simulink subsystem "ParachuteSpatial3DOF"  (R2023b)
settings: Solver=VariableStepAuto  StartTime=0.0  StopTime=10.0  RelTol=1e-3
undefined symbols (not defined in the file): alt
libraries: aerolibatmos2 x1, matrix_library x1, vrlib x1
settings Model: Creator=thatf  LastModifiedBy=thatf

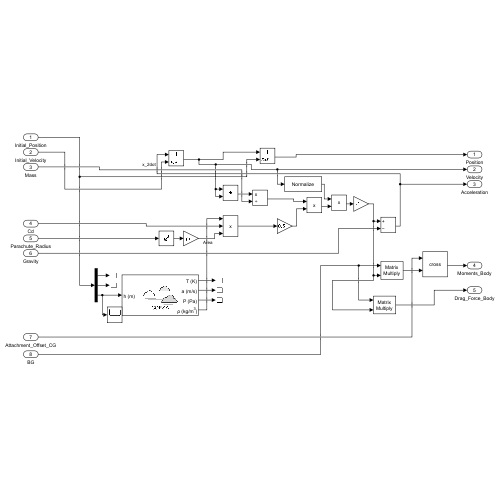
[thumbnail: Simulink's stored preview of the top-level diagram]
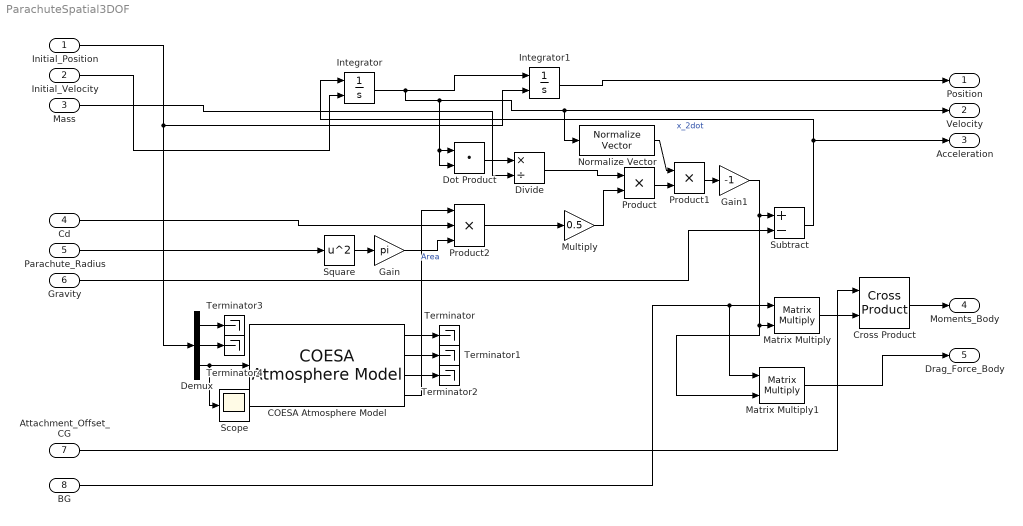
== system ParachuteSpatial3DOF ==
  Initial_Position : Inport
  Initial_Velocity : Inport  Port=2
  Mass : Inport  Port=3
  Cd : Inport  Port=4
  Parachute_Radius : Inport  Port=5
  Gravity : Inport  Port=6
  Attachment_Offset_CG : Inport  Port=7
  BG : Inport  Port=8
  COESA Atmosphere Model : aerolibatmos2/COESA Atmosphere Model  units=Metric (MKS)  spec=1976 COESA-extended U.S. Standard Atmosphere  model=Profile  profile_var=High temperature  profile_percent=1%  profile_alt=5 km (16404 ft)  envelope_var=High temperature  envelope_percent=1%  action=Warning
  Cross Product : matrix_library/Cross Product
  Demux : Demux  Outputs=3
  Divide : Product  Inputs=*/
  Dot Product : DotProduct  OutDataTypeStr=Inherit: Inherit via internal rule
  Gain : Gain  Gain=pi
  Gain1 : Gain  Gain=-1
  Integrator : Integrator  InitialConditionSource=external
  Integrator1 : Integrator  InitialConditionSource=external  InitialCondition=alt
  Matrix Multiply : Product  Multiplication=Matrix(*)
  Matrix Multiply1 : Product  Multiplication=Matrix(*)
  Multiply : Gain  Gain=0.5
  Normalize Vector : vrlib/Utilities/Normalize Vector  maxzero=0
  Product : Product
  Product1 : Product
  Product2 : Product  Inputs=3
  Scope : Scope
  Square : Math  Operator=square
  Subtract : Sum  Inputs=+-
  Terminator{,1..4} (5 alike) : Terminator
  Position : Outport
  Velocity : Outport  Port=2
  Acceleration : Outport  Port=3
  Moments_Body : Outport  Port=4
  Drag_Force_Body : Outport  Port=5
  wires:
  Normalize Vector/1 -> Product1/1
  Subtract/1 -> Integrator/1, Acceleration/1  "x_2dot"
  Divide/1 -> Product/1
  Product/1 -> Product1/2
  Dot Product/1 -> Divide/1
  Integrator/1 -> Integrator1/1, Dot Product/1, Dot Product/2, Normalize Vector/1, Velocity/1
  Gravity/1 -> Subtract/2
  Mass/1 -> Divide/2
  Multiply/1 -> Product/2
  Product2/1 -> Multiply/1
  Cd/1 -> Product2/2
  Square/1 -> Gain/1
  Gain/1 -> Product2/3  "Area"
  Parachute_Radius/1 -> Square/1
  Integrator1/1 -> Position/1
  COESA Atmosphere Model/4 -> Product2/1
  COESA Atmosphere Model/1 -> Terminator/1
  COESA Atmosphere Model/2 -> Terminator1/1
  COESA Atmosphere Model/3 -> Terminator2/1
  Demux/3 -> COESA Atmosphere Model/1, Scope/1
  Demux/1 -> Terminator3/1
  Demux/2 -> Terminator4/1
  Product1/1 -> Gain1/1
  Gain1/1 -> Subtract/1, Matrix Multiply/2, Matrix Multiply1/2
  Attachment_Offset_CG/1 -> Cross Product/1
  Matrix Multiply/1 -> Cross Product/2
  Cross Product/1 -> Moments_Body/1
  BG/1 -> Matrix Multiply/1, Matrix Multiply1/1
  Matrix Multiply1/1 -> Drag_Force_Body/1
  Initial_Velocity/1 -> Integrator/2
  Initial_Position/1 -> Integrator1/2, Demux/1
